simulink model "GovModel02"  (R2014a)
settings: Solver=ode3  StartTime=tstart  StopTime=tstop  FixedStep=dt  RelTol=1e-3
values from neighbouring files (symbols this model uses):
  Dt = 0    [SimulinkGov.m]
  R = 0.05    [SimulinkGov.m]
  T1 = 0.5    [SimulinkGov.m]
  T2 = 3.0    (= 3)    [SimulinkGov.m]
  T3 = 10    [SimulinkGov.m]
settings Model: Creator=mstajcar  LastModifiedBy=MStajcar

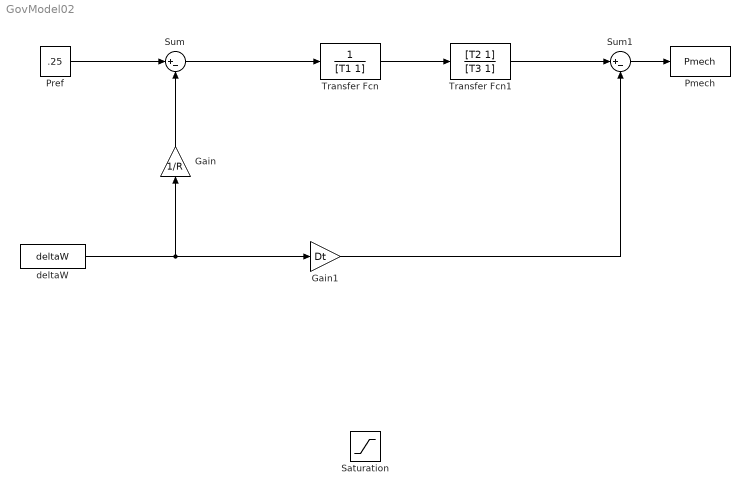
== system GovModel02 ==
  Gain : Gain  Gain=1/R
  Gain1 : Gain  Gain=Dt
  Pmech : ToWorkspace  VariableName=Pmech  SampleTime=-1
  "Pref " : Constant  Value=.25
  Saturation : Saturate  UpperLimit=1  LowerLimit=0
  Sum : Sum  Inputs=|+-
  Sum1 : Sum  Inputs=|+-
  Transfer Fcn : TransferFcn  Denominator=[T1 1]
  Transfer Fcn1 : TransferFcn  Numerator=[T2 1]  Denominator=[T3 1]
  deltaW : FromWorkspace  VariableName=deltaW  SampleTime=0
  wires:
  Sum/1 -> Transfer Fcn/1
  Transfer Fcn1/1 -> Sum1/1
  Gain1/1 -> Sum1/2
  "Pref "/1 -> Sum/1
  Transfer Fcn/1 -> Transfer Fcn1/1
  deltaW/1 -> Gain/1, Gain1/1
  Sum1/1 -> Pmech/1
  Gain/1 -> Sum/2
